simulink model "simulink_disturbio"  (R2021a)
settings: Solver=VariableStepAuto  StartTime=0.0  StopTime=130  RelTol=1e-3
values from neighbouring files (symbols this model uses):
  Ts = tsd/25    (= 0.0072)    [list2_questao_extra.m]
settings Model: Creator=ribei  LastModifiedBy=check
settings SolverCC: AlgebraicLoopSolver=TrustRegion
settings DebuggingCC: UnconnectedInputMsg=none  UnconnectedOutputMsg=none  UnconnectedLineMsg=none  SFMachineParentedDataDiag=warning  ArithmeticOperatorsInVariantConditions=warning
settings ModelReferenceCC: EnableRefExpFcnMdlSchedulingChecks=off
settings SFSimCC: CustomCodeUndefinedFunction=UseInterfaceOnly
settings RTWCC: Description=Generic Real-Time Target
settings CodeAppCC: StateflowObjectComments=on

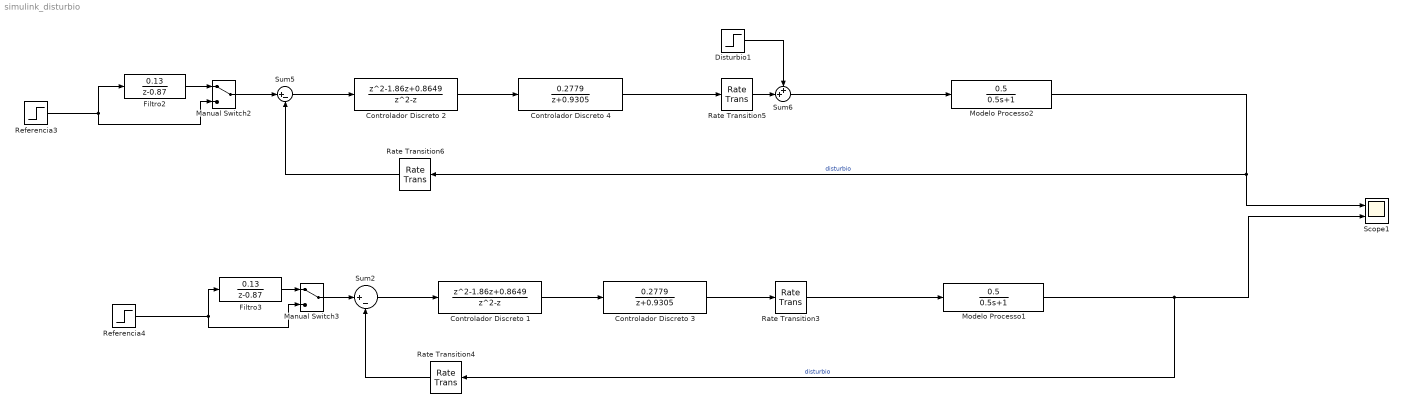
== system simulink_disturbio ==
  Controlador Discreto 1 : DiscreteTransferFcn  Numerator=[1 -1.86 0.8649]  Denominator=[1 -1 0]
  Controlador Discreto 2 : DiscreteTransferFcn  Numerator=[1 -1.86 0.8649]  Denominator=[1 -1 0]
  Controlador Discreto 3 : DiscreteTransferFcn  Numerator=[0.2779]  Denominator=[1 0.9305]
  Controlador Discreto 4 : DiscreteTransferFcn  Numerator=[0.2779]  Denominator=[1 0.9305]
  Disturbio1 : Step  Time=35  SampleTime=Ts  VectorParams1D=off
  Filtro2 : DiscreteTransferFcn  Numerator=[0.13]  Denominator=[1 -0.87]
  Filtro3 : DiscreteTransferFcn  Numerator=[0.13]  Denominator=[1 -0.87]
  Manual Switch2 : ManualSwitch
  Manual Switch3 : ManualSwitch
  Modelo Processo1 : TransferFcn  Numerator=[0.5]  Denominator=[0.5 1]
  Modelo Processo2 : TransferFcn  Numerator=[0.5]  Denominator=[0.5 1]
  Rate Transition3 : RateTransition  Integrity=off  OutPortSampleTimeOpt=Inherit
  Rate Transition4 : RateTransition  OutPortSampleTime=Ts
  Rate Transition5 : RateTransition  Integrity=off  OutPortSampleTimeOpt=Inherit
  Rate Transition6 : RateTransition  OutPortSampleTime=Ts
  Referencia3 : Step  SampleTime=Ts
  Referencia4 : Step  SampleTime=Ts
  Scope1 : Scope  NumInputPorts=2
  Sum2 : Sum  Inputs=|+-
  Sum5 : Sum  Inputs=|+-
  Sum6 : Sum  Inputs=++|
  wires:
  Sum5/1 -> Controlador Discreto 2/1
  Filtro3/1 -> Manual Switch3/1
  Referencia4/1 -> Filtro3/1, Manual Switch3/2
  Filtro2/1 -> Manual Switch2/1
  Manual Switch2/1 -> Sum5/1
  Rate Transition5/1 -> Sum6/2
  Rate Transition6/1 -> Sum5/2
  Modelo Processo2/1 -> Scope1/1, Rate Transition6/1  "disturbio"
  Referencia3/1 -> Filtro2/1, Manual Switch2/2
  Disturbio1/1 -> Sum6/1
  Controlador Discreto 2/1 -> Controlador Discreto 4/1
  Controlador Discreto 4/1 -> Rate Transition5/1
  Sum6/1 -> Modelo Processo2/1
  Rate Transition3/1 -> Modelo Processo1/1
  Controlador Discreto 3/1 -> Rate Transition3/1
  Controlador Discreto 1/1 -> Controlador Discreto 3/1
  Sum2/1 -> Controlador Discreto 1/1
  Modelo Processo1/1 -> Rate Transition4/1, Scope1/2  "disturbio"
  Manual Switch3/1 -> Sum2/1
  Rate Transition4/1 -> Sum2/2
